simulink model "QPTest5"  (R2021a)
settings: Solver=ode45  StartTime=0.0  StopTime=20  FixedStep=Control_timestep  RelTol=1e-3  AbsTol=1e-6
undefined symbols (not defined in the file): Matlab_version, NXMotion, NXMotion_controltimestep, NXMotion_model, NXMotion_model_n, NXMotion_n, NXMotion_solution, NXMotion_solution_n, Plant_inputs_num, Plant_outputs_num
libraries: simulink x1
(part 3 of 3)

== matlab function QPTest5/MATLAB Function14 ==
  data: X1 input; X2 input; X3 input; X4 input; X5 input; X6 input; B1 input; B2 input; B3 input; B4 input; B5 input; B6 input; F1 input; F2 input; F3 input; F4 input; F5 input; F6 input; q1 input; q2 input; q3 input; q4 input; q5 input; q6 input; q7 input; q8 input; q9 input; q10 input; q11 input; q12 input; qdot1 input; qdot2 input; qdot3 input; qdot4 input; qdot5 input; qdot6 input; qdot7 input; qdot8 input; qdot9 input; qdot10 input; qdot11 input; qdot12 input; qddot1 input; qddot2 input; qddot3 input; qddot4 input; qddot5 input; qddot6 input; qddot7 input; qddot8 input; qddot9 input; qddot10 input; qddot11 input; qddot12 input; Xdot1 input; Xdot2 input; Xdot3 input; Xdot4 input; Xdot5 input; Xdot6 input; t_before input; X_act output; Xdot_act output; F_act output; q output; qdot output; qddot output
function [X_act, Xdot_act, F_act, q, qdot, qddot] = Integrator( ...
    X1, X2, X3, X4, X5, X6, ...
    B1, B2, B3, B4, B5, B6, ...
    F1, F2, F3, F4, F5, F6, ...
    q1, q2, q3, q4, q5, q6, q7, q8, q9, q10, q11, q12, ...
    qdot1, qdot2, qdot3, qdot4, qdot5, qdot6, qdot7, qdot8, qdot9, qdot10, qdot11, qdot12, ...
    qddot1, qddot2, qddot3, qddot4, qddot5, qddot6, qddot7, qddot8, qddot9, qddot10, qddot11, qddot12, ...
    Xdot1, Xdot2, Xdot3, Xdot4, Xdot5, Xdot6, ...
    t_before)

    %% -------------------------------------------------
    % 0. 固定输出尺寸
    % --------------------------------------------------
    X_act    = zeros(6,1);
    Xdot_act = zeros(6,1);
    F_act    = zeros(6,1);
    q        = zeros(13,1);
    qdot     = zeros(13,1);
    qddot    = zeros(13,1);

    %% -------------------------------------------------
    % 0.1 数据记录设置
    % --------------------------------------------------
    coder.extrinsic('assignin', 'evalin');

    persistent log_is_init
    persistent log_k
    persistent log_t_last
    persistent log_next_t
    persistent log_saved_final
    persistent log_overflow

    persistent log_t
    persistent log_X_act
    persistent log_Xdot_act
    persistent log_F_act
    persistent log_q
    persistent log_qdot
    persistent log_qddot

    % --------------------------------------------------
    % 强制将 Clock 输入整理为标量时间
    % --------------------------------------------------
    t_vec = t_before(:);
    t = t_vec(1);

    % 记录采样周期，建议与你的控制周期一致
    dt_log = 1.0e-3;      % s

    % 当前仿真时长。如果你的仿真不是 10 s，在这里改。
    % 如果你当前仿真是 20 s，请保留 20.0。
    t_stop_save = 20.0;   % s

    % 最大记录点数。
    % 20 s @ 1 kHz = 20000 点。
    % 这里留一点余量。
    maxLogN = 30000;

    % 自动保存间隔。
    % 1000 点约等于每 1 s 自动保存一次。
    autosave_every = 1000;

    % 初始化或检测到新一轮仿真开始
    if isempty(log_is_init)
        log_is_init     = true;
        log_k           = 0;
        log_t_last      = -1.0e99;
        log_next_t      = 0.0;
        log_saved_final = false;
        log_overflow    = false;

        log_t        = zeros(1, maxLogN);
        log_X_act    = zeros(6, maxLogN);
        log_Xdot_act = zeros(6, maxLogN);
        log_F_act    = zeros(6, maxLogN);
        log_q        = zeros(13, maxLogN);
        log_qdot     = zeros(13, maxLogN);
        log_qddot    = zeros(13, maxLogN);
    end

    % 如果仿真时间回跳，说明重新开始了一次仿真，清空日志
    if t < log_t_last - 1.0e-12
        log_k           = 0;
        log_next_t      = 0.0;
        log_saved_final = false;
        log_overflow    = false;

        log_t(:)        = 0.0;
        log_X_act(:)    = 0.0;
        log_Xdot_act(:) = 0.0;
        log_F_act(:)    = 0.0;
        log_q(:)        = 0.0;
        log_qdot(:)     = 0.0;
        log_qddot(:)    = 0.0;
    end

    log_t_last = t;

    %% -------------------------------------------------
    % 1. 与 Parameters() 一致的几何参数
    %
    % 如果 Parameters() 中 A、B、Theta0 后续修改，
    % 这里也必须同步修改。
    % --------------------------------------------------
    A0 = [
         415.6893,  396.4603, 1107;
        -415.6893,  396.4603, 1107;
        -551.1893,  161.7674, 1107;
        -135.5000, -558.2276, 1107;
         135.5000, -558.2276, 1107;
         551.1893,  161.7674, 1107
    ];

    B0 = [
         196.5673,  921.7786, 132;
        -196.5673,  921.7786, 132;
        -896.5673, -290.6569, 132;
        -700.0000, -631.1216, 132;
         700.0000, -631.1216, 132;
         896.5673, -290.6569, 132
    ];

    Theta0_abs = [
          0.0000;
         30.0000;
          0.0000;
        -120.0000;
          0.0000;
        150.0000;
          0.0000
    ];

    %% -------------------------------------------------
    % 2. 计算 Stewart 初始绝对电缸长度 L0
    %
    % NX 输出的是 stroke，因此控制器所需绝对长度为：
    %   l_i = L0_i + stroke_i
    % --------------------------------------------------
    dAB = A0 - B0;

    L0 = zeros(6,1);
    for i = 1:6
        L0(i) = sqrt( ...
            dAB(i,1)*dAB(i,1) + ...
            dAB(i,2)*dAB(i,2) + ...
            dAB(i,3)*dAB(i,3));
    end

    %% -------------------------------------------------
    % 3. 末端实际位姿、速度、力
    % --------------------------------------------------
    rad2deg = 180.0 / pi;

    % 末端位置，单位 mm
    X_act(1) = safe_scalar_local(X1);
    X_act(2) = safe_scalar_local(X2);
    X_act(3) = safe_scalar_local(X3);

    % 末端姿态角，单位 deg
    X_act(4) = safe_scalar_local(X4) * rad2deg;
    X_act(5) = safe_scalar_local(X5) * rad2deg;
    X_act(6) = safe_scalar_local(X6) * rad2deg;

    % 末端线速度，单位 mm/s
    Xdot_act(1) = safe_scalar_local(Xdot1);
    Xdot_act(2) = safe_scalar_local(Xdot2);
    Xdot_act(3) = safe_scalar_local(Xdot3);

    % 末端姿态速度，单位 deg/s
    Xdot_act(4) = safe_scalar_local(Xdot4) * rad2deg;
    Xdot_act(5) = safe_scalar_local(Xdot5) * rad2deg;
    Xdot_act(6) = safe_scalar_local(Xdot6) * rad2deg;

    % 力/力矩
    F_act(1) = safe_scalar_local(F1);
    F_act(2) = safe_scalar_local(F2);
    F_act(3) = safe_scalar_local(F3);
    F_act(4) = safe_scalar_local(F4);
    F_act(5) = safe_scalar_local(F5);
    F_act(6) = safe_scalar_local(F6);

    %% -------------------------------------------------
    % 4. NX 输出的相对驱动量
    % --------------------------------------------------
    stroke = zeros(6,1);
    stroke(1) = safe_scalar_local(q1);
    stroke(2) = safe_scalar_local(q2);
    stroke(3) = safe_scalar_local(q3);
    stroke(4) = safe_scalar_local(q4);
    stroke(5) = safe_scalar_local(q5);
    stroke(6) = safe_scalar_local(q6);

    delta_theta = zeros(7,1);
    delta_theta(1) = safe_scalar_local(q7);
    delta_theta(2) = safe_scalar_local(q8);
    delta_theta(3) = safe_scalar_local(q9);
    delta_theta(4) = safe_scalar_local(q10);
    delta_theta(5) = safe_scalar_local(q11);
    delta_theta(6) = safe_scalar_local(q12);
    delta_theta(7) = 0.0;

    %% -------------------------------------------------
    % 5. 转换为控制器需要的绝对 q
    % --------------------------------------------------
    q(1:6) = L0 + stroke;

    delta_theta = delta_theta * rad2deg;
    
    q(7:13) = Theta0_abs + delta_theta;

    q(13) = Theta0_abs(7);

    %% -------------------------------------------------
    % 6. 速度转换
    % --------------------------------------------------
    qdot(1) = safe_scalar_local(qdot1);
    qdot(2) = safe_scalar_local(qdot2);
    qdot(3) = safe_scalar_local(qdot3);
    qdot(4) = safe_scalar_local(qdot4);
    qdot(5) = safe_scalar_local(qdot5);
    qdot(6) = safe_scalar_local(qdot6);

    qdot(7)  = safe_scalar_local(qdot7)  * rad2deg;
    qdot(8)  = safe_scalar_local(qdot8)  * rad2deg;
    qdot(9)  = safe_scalar_local(qdot9)  * rad2deg;
    qdot(10) = safe_scalar_local(qdot10) * rad2deg;
    qdot(11) = safe_scalar_local(qdot11) * rad2deg;
    qdot(12) = safe_scalar_local(qdot12) * rad2deg;

    % 第 7 机械臂关节固定
    qdot(13) = 0.0;

    %% -------------------------------------------------
    % 7. 加速度转换
    %
    % 注意：
    %   这里的 qddot 是 NX 直接输出的原始加速度通道。
    %   后续保存到 Integrator_Log.qddot 时，不再直接使用该通道，
    %   而是在 local_save_integrator_log 中由 qdot 对 t 数值微分得到。
    %   该原始通道会保存为 Integrator_Log.qddot_raw。
    % --------------------------------------------------
    qddot(1) = safe_scalar_local(qddot1);
    qddot(2) = safe_scalar_local(qddot2);
    qddot(3) = safe_scalar_local(qddot3);
    qddot(4) = safe_scalar_local(qddot4);
    qddot(5) = safe_scalar_local(qddot5);
    qddot(6) = safe_scalar_local(qddot6);

    qddot(7)  = safe_scalar_local(qddot7)  * rad2deg;
    qddot(8)  = safe_scalar_local(qddot8)  * rad2deg;
    qddot(9)  = safe_scalar_local(qddot9)  * rad2deg;
    qddot(10) = safe_scalar_local(qddot10) * rad2deg;
    qddot(11) = safe_scalar_local(qddot11) * rad2deg;
    qddot(12) = safe_scalar_local(qddot12) * rad2deg;

    % 第 7 机械臂关节固定
    qddot(13) = 0.0;

    %% -------------------------------------------------
    % 8. 保留 B1~B6，避免误以为漏接
    % --------------------------------------------------
    unused_B_sum = B1 + B2 + B3 + B4 + B5 + B6; %#ok<NASGU>

    %% -------------------------------------------------
    % 9. 记录输出数据，并保存为 MAT 文件
    %
    % 记录内容：
    %   Integrator_Log.t
    %   Integrator_Log.X_act
    %   Integrator_Log.Xdot_act
    %   Integrator_Log.F_act
    %   Integrator_Log.q
    %   Integrator_Log.qdot
    %   Integrator_Log.qddot
    %   Integrator_Log.qddot_raw
    %
    % 注意：
    %   Integrator_Log.qddot 由 qdot 对 t 数值微分得到；
    %   Integrator_Log.qddot_raw 为 NX 直接输出的原始 qddot 通道。
    %   文件保存到 MATLAB 当前工作路径。
    % --------------------------------------------------
    do_log = false;

    if t + 1.0e-12 >= log_next_t
        do_log = true;
        log_next_t = t + dt_log;
    end

    if do_log
        if log_k < maxLogN
            log_k = log_k + 1;

            log_t(log_k)          = t;
            log_X_act(:,log_k)    = X_act;
            log_Xdot_act(:,log_k) = Xdot_act;
            log_F_act(:,log_k)    = F_act;
            log_q(:,log_k)        = q;
            log_qdot(:,log_k)     = qdot;
            log_qddot(:,log_k)    = qddot;
        else
            log_overflow = true;
        end
    end

    do_save = false;

    % 周期性自动保存，避免仿真中途停止时数据完全丢失
    if log_k > 0
        if mod(log_k, autosave_every) == 0
            do_save = true;
        end
    end

    % 到达仿真末端时最终保存一次
    if ~log_saved_final
        if t >= t_stop_save - 0.5 * dt_log
            do_save = true;
            log_saved_final = true;
        end
    end

    if do_save
        local_save_integrator_log( ...
            log_k, dt_log, t_stop_save, log_overflow, ...
            log_t, log_X_act, log_Xdot_act, log_F_act, ...
            log_q, log_qdot, log_qddot);
    end

end

%% ========================================================================
%                    保存 Integrator 记录数据到 MAT 文件
% ========================================================================

function local_save_integrator_log( ...
    log_k, dt_log, t_stop_save, log_overflow, ...
    log_t, log_X_act, log_Xdot_act, log_F_act, ...
    log_q, log_qdot, log_qddot)

% --------------------------------------------------
% Integrator_Log 数据结构说明
%
% Integrator_Log 是保存 NX Motion Plant 输出反馈数据的 struct。
%
% 字段说明：
%   n
%       类型：double 标量
%       含义：实际记录的数据点数。
%
%   dt_log
%       类型：double 标量
%       含义：数据记录采样周期，单位 s。
%
%   t_stop_save
%       类型：double 标量
%       含义：设定的仿真终止保存时间，单位 s。
%
%   overflow
%       类型：logical 标量
%       含义：记录数组是否超过最大预分配长度。
%
%   t
%       类型：1 x n double
%       含义：每个记录点对应的仿真时间，单位 s。
%
%   X_act
%       类型：6 x n double
%       含义：末端实际位姿。
%       单位：[mm; mm; mm; deg; deg; deg]。
%
%   Xdot_act
%       类型：6 x n double
%       含义：末端实际速度。
%       单位：[mm/s; mm/s; mm/s; deg/s; deg/s; deg/s]。
%
%   F_act
%       类型：6 x n double
%       含义：末端实际接触力/力矩反馈。
%       单位：[N; N; N; Nmm_or_Nm; Nmm_or_Nm; Nmm_or_Nm]。
%
%   q
%       类型：13 x n double
%       含义：系统广义坐标反馈。
%       q(1:6) 为 Stewart 六个电缸绝对长度，单位 mm；
%       q(7:13) 为机械臂七个关节角，单位 deg。
%
%   qdot
%       类型：13 x n double
%       含义：系统广义速度反馈。
%       qdot(1:6) 单位 mm/s；
%       qdot(7:13) 单位 deg/s。
%
%   qddot
%       类型：13 x n double
%       含义：系统广义加速度反馈，由 qdot 对 t 数值微分得到。
%       qddot(1:6) 单位 mm/s^2；
%       qddot(7:13) 单位 deg/s^2。
%
%   qddot_raw
%       类型：13 x n double
%       含义：NX/Motion 直接输出的原始 qddot 通道，仅用于对比检查。
%
%   units
%       类型：struct
%       含义：上述主要变量的单位说明。
% --------------------------------------------------

    coder.extrinsic('assignin', 'evalin');

    assignin('base', 'tmp_Integrator_Log_n',           log_k);
    assignin('base', 'tmp_Integrator_Log_dt_log',      dt_log);
    assignin('base', 'tmp_Integrator_Log_t_stop_save', t_stop_save);
    assignin('base', 'tmp_Integrator_Log_overflow',    log_overflow);

    assignin('base', 'tmp_Integrator_Log_t',           log_t);
    assignin('base', 'tmp_Integrator_Log_X_act',       log_X_act);
    assignin('base', 'tmp_Integrator_Log_Xdot_act',    log_Xdot_act);
    assignin('base', 'tmp_Integrator_Log_F_act',       log_F_act);
    assignin('base', 'tmp_Integrator_Log_q',           log_q);
    assignin('base', 'tmp_Integrator_Log_qdot',        log_qdot);
    assignin('base', 'tmp_Integrator_Log_qddot_raw',   log_qddot);

    evalin('base', [ ...
        'idx = 1:tmp_Integrator_Log_n;' ...
        'Integrator_Log = struct();' ...
        'Integrator_Log.n = tmp_Integrator_Log_n;' ...
        'Integrator_Log.dt_log = tmp_Integrator_Log_dt_log;' ...
        'Integrator_Log.t_stop_save = tmp_Integrator_Log_t_stop_save;' ...
        'Integrator_Log.overflow = tmp_Integrator_Log_overflow;' ...
        'Integrator_Log.t = tmp_Integrator_Log_t(idx);' ...
        'Integrator_Log.X_act = tmp_Integrator_Log_X_act(:,idx);' ...
        'Integrator_Log.Xdot_act = tmp_Integrator_Log_Xdot_act(:,idx);' ...
        'Integrator_Log.F_act = tmp_Integrator_Log_F_act(:,idx);' ...
        'Integrator_Log.q = tmp_Integrator_Log_q(:,idx);' ...
        'Integrator_Log.qdot = tmp_Integrator_Log_qdot(:,idx);' ...
        'Integrator_Log.qddot_raw = tmp_Integrator_Log_qddot_raw(:,idx);' ...
        'Integrator_Log.qddot = zeros(size(Integrator_Log.qdot));' ...
        'if Integrator_Log.n >= 2;' ...
        'for ii = 1:size(Integrator_Log.qdot,1);' ...
        'Integrator_Log.qddot(ii,:) = gradient(Integrator_Log.qdot(ii,:), Integrator_Log.t);' ...
        'end;' ...
        'end;' ...
        'Integrator_Log.units = struct();' ...
        'Integrator_Log.units.t = ''s'';' ...
        'Integrator_Log.units.X_act = ''[mm; mm; mm; deg; deg; deg]'';' ...
        'Integrator_Log.units.Xdot_act = ''[mm/s; mm/s; mm/s; deg/s; deg/s; deg/s]'';' ...
        'Integrator_Log.units.F_act = ''[N; N; N; Nmm_or_Nm; Nmm_or_Nm; Nmm_or_Nm]'';' ...
        'Integrator_Log.units.q = ''[Stewart mm x6; Arm deg x7]'';' ...
        'Integrator_Log.units.qdot = ''[Stewart mm/s x6; Arm deg/s x7]'';' ...
        'Integrator_Log.units.qddot = ''computed by gradient(qdot,t): [Stewart mm/s^2 x6; Arm deg/s^2 x7]'';' ...
        'Integrator_Log.units.qddot_raw = ''raw NX/Motion qddot channel: [Stewart mm/s^2 x6; Arm deg/s^2 x7]'';' ...
        'save(''NXPlant_Integrator_Log.mat'', ''Integrator_Log'');' ...
        'clear idx ii tmp_Integrator_Log_n tmp_Integrator_Log_dt_log tmp_Integrator_Log_t_stop_save tmp_Integrator_Log_overflow ' ...
        'tmp_Integrator_Log_t tmp_Integrator_Log_X_act tmp_Integrator_Log_Xdot_act tmp_Integrator_Log_F_act ' ...
        'tmp_Integrator_Log_q tmp_Integrator_Log_qdot tmp_Integrator_Log_qddot_raw;' ...
    ]);

end

%% ========================================================================
%                    NaN / Inf 保护
% ========================================================================

function y = safe_scalar_local(x)
% NaN / Inf 保护，避免异常值直接进入控制器。

    if isfinite(x)
        y = x;
    else
        y = 0.0;
    end

end

== matlab function QPTest5/MATLAB Function1 ==
  data: A output; B output; XB output; P0 output; dh output; Theta0 output
function [A, B, XB, P0, dh, Theta0] = Parameters()

%   A       6x3  Stewart 上平台 6 个 A 铰链点坐标，单位 mm
%   B       6x3  Stewart 下平台 6 个 B 铰链点坐标，单位 mm
%   XB      3x1  机械臂基座原点初始位置坐标，单位 mm
%   P0      3x1  Stewart 上平台中心初始位置坐标，单位 mm
%   dh      7x4  机械臂 MDH 参数 [a, d, alpha, theta_offset]
%                其中：
%                a, d 单位为 mm
%                alpha, theta_offset 单位为 deg
%   Theta0  7x1  机械臂 7 个关节在打磨初始位置的角度，单位 deg
%
% 单位约定：
%   长度：mm
%   角度：deg
%
% 当前系统状态量 q 的顺序：
%
%   q = [L0; Theta0]
%     = [l1; l2; l3; l4; l5; l6; theta1; theta2; ...; theta7]
%
% 其中：
%   q(1:6)    为 Stewart 6 个电缸长度，单位 mm；
%   q(7:13)   为机械臂 7 个关节位置，单位 deg；
%   q(13)     为机械臂第 7 关节，当前固定。

    % -----------------------------
    % 0. 固定输出尺寸，便于 Simulink 推断
    % -----------------------------
    A      = zeros(6,3);
    B      = zeros(6,3);
    XB     = zeros(3,1);
    P0     = zeros(3,1);
    dh     = zeros(7,4);
    Theta0 = zeros(7,1);

    % -----------------------------
    % Stewart 上平台 A 铰链点坐标
    % 单位：mm
    % -----------------------------
    A = [
         415.6893,  396.4603, 1107;
        -415.6893,  396.4603, 1107;
        -551.1893,  161.7674, 1107;
        -135.5000, -558.2276, 1107;
         135.5000, -558.2276, 1107;
         551.1893,  161.7674, 1107
    ];

    % -----------------------------
    % Stewart 下平台 B 铰链点坐标
    % 单位：mm
    % -----------------------------
    B = [
         196.5673,  921.7786, 132;
        -196.5673,  921.7786, 132;
        -896.5673, -290.6569, 132;
        -700.0000, -631.1216, 132;
         700.0000, -631.1216, 132;
         896.5673, -290.6569, 132
    ];

    % -----------------------------
    % 机械臂基座原点初始位置坐标
    % 单位：mm
    % -----------------------------
    XB = [
        0;
        0;
        1224
    ];

    % -----------------------------
    % Stewart 上平台中心初始位置坐标
    % 单位：mm
    % -----------------------------
    P0 = [
        0;
        0;
        1107
    ];

    % -----------------------------
    % 机械臂 MDH 参数
    % 每行格式：[a, d, alpha, theta_offset]
    %
    % a, d 单位：mm
    % alpha, theta_offset 单位：deg
    %
    % 第 7 行仍然保留，因为它描述第 7 固定关节
    % 以及末端工具安装位姿。
    % -----------------------------
    dh = [
         0.0000,       666.0000,   0.0000,   0.0000;
         0.0000,         0.0000, -90.0000,   0.0000;
         0.0000,       632.0000,  90.0000,   0.0000;
         82.5*2,         0.0000,  90.0000,   0.0000;
        -82.5*2,       768.0000, -90.0000,   0.0000;
         0.0000,         0.0000,  90.0000,   0.0000;
         176.0000,     214.0000,  90.0000,   0.0000
    ];

    % -----------------------------
    % 机械臂 7 个关节在打磨初始位置的角度
    % 单位：deg
    %
    % 其中第 7 关节固定，但仍放入 Theta0，
    % 使 q(7:13) 对应机械臂 7 个关节位置。
    % -----------------------------
    Theta0 = [
          0.0000;
         30.0000;
          0.0000;
        -120.0000;
          0.0000;
        150.0000;
          0.0000
    ];

end
